simulink model "MODEL_FULL_SYSTEM_MUTUAL"  (Simulink 7.8)
settings: Solver=ode1  StartTime=0.0  StopTime=inf  FixedStep=Ts  MaxStep=1e-3  RelTol=1e-3
PostLoadFcn:
  | Ts=80e-6; relays_settings_init;
InitFcn:
  | Ts=80e-6; relays_settings_init;
values from neighbouring files (symbols this model uses):
  relay_sets = xlsread('relay_settings_10272015.xlsx')    [relays_settings_init.m]
undefined symbols (not defined in the file or in its folder): dfilt, DiscIntNeverNeededParam, fdesignblkfcn, gcbh, Left, opmodbus_cb, ph, Right, type, V, X
libraries: simulink x72, modbus_lib x40, cables_lib x36, rtio_opalrt_common x21, rtlab x20, transformer_lib x13, dynamic_load_lib x12, powerlib x6, simulink_extras x6, ssn_lib x5, discretizing x4, rteventslib x4
(part 4 of 7)

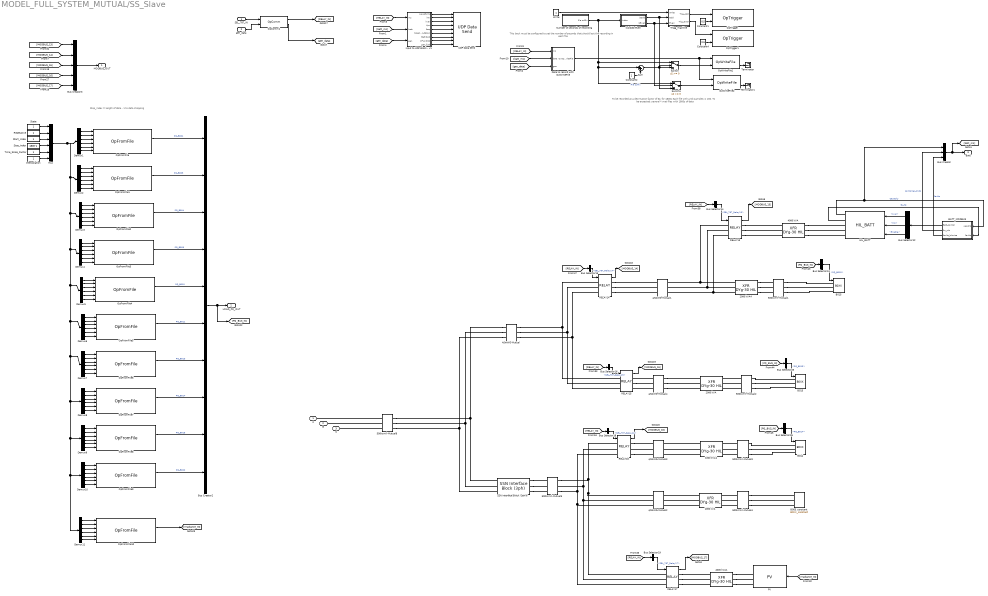
== system MODEL_FULL_SYSTEM_MUTUAL/SS_Slave ==
  note: Stop_index = length of data - 1 to data chopping
  note: This bock must be configured to set the number of
      | seconds that should last the recording in each file
  note: To be recorded at a decimation factor of 62,   for 1800s each file with a Nb samples = 200.
      | To be expected: several *.mat files with 1800s of data
  SEL_787_IN : Inport
  gen_data : Inport  Port=2
  1000 kVA : transformer_lib/XFR DYg-30 HIL  Rating=1000  Vp=4160  Vs=460  Z=5.18  XR=2.5
  1000 kVA1 : transformer_lib/XFR DYg-30 HIL  Rating=1000  Vp=4160  Vs=216  Z=5.18  XR=2.5
  2000 kVA : transformer_lib/XFR DYg-30 HIL  Rating=2000  Vp=4160  Vs=216  Z=5.18  XR=2.5
  2000 kVA4 : transformer_lib/XFR DYg-30 HIL  Rating=2000  Vp=4160  Vs=216  Z=5.18  XR=2.5
  4/0AWG-Mutual : cables_lib/4//0AWG-Mutual  length=20  par_sets=1  ratio=3
  4/0AWG-Mutual{1..4} (4 alike) : cables_lib/4//0AWG-Mutual  length=51  par_sets=1  ratio=3
  4000 kVA : transformer_lib/XFR DYg-30 HIL  Rating=4000  Vp=2047  Vs=4160  Z=6.37  XR=3.5
  4000 kVA1 : transformer_lib/XFR DYg-30 HIL  Rating=4000  Vp=2047  Vs=4160  Z=6.37  XR=3.5
  500kcmil-Mutual{1..4} (4 alike) : cables_lib/500kcmil-Mutual  length=25  par_sets=1  ratio=3
  500kcmil-Mutual5 : cables_lib/500kcmil-Mutual  length=50  par_sets=1  ratio=3
  500kcmil-Mutual8 : cables_lib/500kcmil-Mutual  length=50  par_sets=1  ratio=3
  B003_constant : dynamic_load_lib/B0XX_constant  v=460  kVA=60  pf=0.9
  B013 : dynamic_load_lib/B0XX  V=208  P_Scale=2  Q_Scale=2
  B014 : dynamic_load_lib/B0XX  V=208  P_Scale=1  Q_Scale=1
  B015 : dynamic_load_lib/B0XX  V=208  P_Scale=2  Q_Scale=2
  BATT_MODBUS : Subsystem
  Bus Creator : BusCreator  Inputs=3
  Bus Creator2 : BusCreator  Inputs=10
  Bus Creator3 : BusCreator  Inputs=5
  Bus Selector12 : BusSelector  OutputSignals=kvar,kW,Enable
  Bus Selector14 : BusSelector  OutputSignals=SEL_787_Relay13
  Bus Selector15 : BusSelector  OutputSignals=SEL_787_Relay14
  Bus Selector16 : BusSelector  OutputSignals=SEL_787_Relay15
  Bus Selector18 : BusSelector  OutputSignals=SEL_787_Relay16
  Bus Selector19 : BusSelector  OutputSignals=SEL_787_Relay17
  Bus Selector24 : BusSelector  OutputSignals=PQ_B015
  Bus Selector25 : BusSelector  OutputSignals=PQ_B013
  Bus Selector26 : BusSelector  OutputSignals=PQ_B014
  Constant1 : Constant  Value=0.5
  Constant2 : Constant
  Constant4 : Constant  Value=0.5
  Data to record with OpWriteFile : Subsystem
  Demux{1..11} (11 alike) : Demux  Outputs=6
  HIL_BATT : Batt_lib/HIL_BATT
  Input to UDP Block - v1 : Subsystem
  "Interpolation " : Constant
  Mux : Mux  Inputs=6
  Number of seconds of recording : Subsystem  mask{time_s=1800}
      mask prompts: time_s "Time in seconds"
      mask help: Set the number of seconds that should last the recording in each file.
  OpComm1 : rtlab/OpComm  nbport=2  groupe_acq=1  subsys_rate=0  st=0  Synchronization=on  Interpolation=on  Threshold=1.0  Missed_Data=off  Sim_Time=off  Samples=off  dynSigOut=off  from_console=0  warning_done=off  writeOpCommFile=off  Offset=off
  OpFromFile : rtlab/DataLogging/OpFromFile  filename_mode=Static (same filename all the time)  reload_mode=Next time model is paused (Real-Time)  init_file_id=0  filename=B001.mat  rtpath='./'  nrtpath='.\'  sample_time=0
  OpFromFile1 : rtlab/DataLogging/OpFromFile  filename_mode=Static (same filename all the time)  reload_mode=Next time model is paused (Real-Time)  init_file_id=0  filename=B003.mat  rtpath='./'  nrtpath='.\'  sample_time=0
  OpFromFile10 : rtlab/DataLogging/OpFromFile  filename_mode=Static (same filename all the time)  reload_mode=Next time model is paused (Real-Time)  init_file_id=0  filename=irradiance_data.mat  rtpath='./'  nrtpath='.\'  sample_time=Ts
  OpFromFile2 : rtlab/DataLogging/OpFromFile  filename_mode=Static (same filename all the time)  reload_mode=Next time model is paused (Real-Time)  init_file_id=0  filename=B004.mat  rtpath='./'  nrtpath='.\'  sample_time=0
  OpFromFile3 : rtlab/DataLogging/OpFromFile  filename_mode=Static (same filename all the time)  reload_mode=Next time model is paused (Real-Time)  init_file_id=0  filename=B009.mat  rtpath='./'  nrtpath='.\'  sample_time=0
  OpFromFile4 : rtlab/DataLogging/OpFromFile  filename_mode=Static (same filename all the time)  reload_mode=Next time model is paused (Real-Time)  init_file_id=0  filename=B010.mat  rtpath='./'  nrtpath='.\'  sample_time=0
  OpFromFile5 : rtlab/DataLogging/OpFromFile  filename_mode=Static (same filename all the time)  reload_mode=Next time model is paused (Real-Time)  init_file_id=0  filename=B011.mat  rtpath='./'  nrtpath='.\'  sample_time=0
  OpFromFile6 : rtlab/DataLogging/OpFromFile  filename_mode=Static (same filename all the time)  reload_mode=Next time model is paused (Real-Time)  init_file_id=0  filename=B013.mat  rtpath='./'  nrtpath='.\'  sample_time=0
  OpFromFile7 : rtlab/DataLogging/OpFromFile  filename_mode=Static (same filename all the time)  reload_mode=Next time model is paused (Real-Time)  init_file_id=0  filename=B014.mat  rtpath='./'  nrtpath='.\'  sample_time=0
  OpFromFile8 : rtlab/DataLogging/OpFromFile  filename_mode=Static (same filename all the time)  reload_mode=Next time model is paused (Real-Time)  init_file_id=0  filename=B015.mat  rtpath='./'  nrtpath='.\'  sample_time=0
  OpFromFile9 : rtlab/DataLogging/OpFromFile  filename_mode=Static (same filename all the time)  reload_mode=Next time model is paused (Real-Time)  init_file_id=0  filename=B022.mat  rtpath='./'  nrtpath='.\'  sample_time=0
  OpTrigger : rtlab/DataLogging/OpTrigger  Trig_Type=TRIGGER SIGNAL >= TRIGGER LEVEL  Trig_Offset=0  Acq_Group=28
  OpTrigger1 : rtlab/DataLogging/OpTrigger  Trig_Type=TRIGGER SIGNAL >= TRIGGER LEVEL  Trig_Offset=0  Acq_Group=29
  OpWriteFile1 : rtlab/DataLogging/OpWriteFile  Static_File=off  varname=recVar  Filename=A_FILE_RECORDED_o.mat  rtpath='./'  nrtpath='.\'  Acq_Group=28  file_size=200000000  write_offline=off  Sim_Mode=off  Nb_Samples=200  Buffer_size=0
      settings: Decimation=62
  OpWriteFile2 : rtlab/DataLogging/OpWriteFile  Static_File=off  varname=recVar  Filename=A_FILE_RECORDED_e.mat  rtpath='./'  nrtpath='.\'  Acq_Group=29  file_size=200000000  write_offline=on  Sim_Mode=off  Nb_Samples=200  Buffer_size=0
      settings: Decimation=62
  PV : PV_lib/PV  max_power=4e6  VacRMS=1200  VacRMS_limit_pu=[1.15 0.85]
  RELAY13 : modbus_lib/RELAY  Ts=Ts
      link override Three-Phase V-I Measurement/Model/VI/Ia: GotoTag=LibraryTag_Ia
      link override Three-Phase V-I Measurement/Model/VI/Ib: GotoTag=LibraryTag_Ib
      link override Three-Phase V-I Measurement/Model/VI/Ic: GotoTag=LibraryTag_Ic
      link override Three-Phase V-I Measurement/Model/VI/Va: GotoTag=LibraryTag_Va
      link override Three-Phase V-I Measurement/Model/VI/Vb: GotoTag=LibraryTag_Vb
      link override Three-Phase V-I Measurement/Model/VI/Vc: GotoTag=LibraryTag_Vc
      link override Three-Phase V-I Measurement1/Model/VI/Ia: GotoTag=LibraryTag_Ia
      link override Three-Phase V-I Measurement1/Model/VI/Ib: GotoTag=LibraryTag_Ib
      link override Three-Phase V-I Measurement1/Model/VI/Ic: GotoTag=LibraryTag_Ic
      link override Three-Phase V-I Measurement1/Model/VI/Va: GotoTag=LibraryTag_Va
      link override Three-Phase V-I Measurement1/Model/VI/Vb: GotoTag=LibraryTag_Vb
      link override Three-Phase V-I Measurement1/Model/VI/Vc: GotoTag=LibraryTag_Vc
  RELAY14 : modbus_lib/RELAY  Ts=Ts
      link override Three-Phase V-I Measurement/Model/VI/Ia: GotoTag=LibraryTag_Ia
      link override Three-Phase V-I Measurement/Model/VI/Ib: GotoTag=LibraryTag_Ib
      link override Three-Phase V-I Measurement/Model/VI/Ic: GotoTag=LibraryTag_Ic
      link override Three-Phase V-I Measurement/Model/VI/Va: GotoTag=LibraryTag_Va
      link override Three-Phase V-I Measurement/Model/VI/Vb: GotoTag=LibraryTag_Vb
      link override Three-Phase V-I Measurement/Model/VI/Vc: GotoTag=LibraryTag_Vc
      link override Three-Phase V-I Measurement1/Model/VI/Ia: GotoTag=LibraryTag_Ia
      link override Three-Phase V-I Measurement1/Model/VI/Ib: GotoTag=LibraryTag_Ib
      link override Three-Phase V-I Measurement1/Model/VI/Ic: GotoTag=LibraryTag_Ic
      link override Three-Phase V-I Measurement1/Model/VI/Va: GotoTag=LibraryTag_Va
      link override Three-Phase V-I Measurement1/Model/VI/Vb: GotoTag=LibraryTag_Vb
      link override Three-Phase V-I Measurement1/Model/VI/Vc: GotoTag=LibraryTag_Vc
  RELAY15 : modbus_lib/RELAY  Ts=Ts
      link override Three-Phase V-I Measurement/Model/VI/Ia: GotoTag=LibraryTag_Ia
      link override Three-Phase V-I Measurement/Model/VI/Ib: GotoTag=LibraryTag_Ib
      link override Three-Phase V-I Measurement/Model/VI/Ic: GotoTag=LibraryTag_Ic
      link override Three-Phase V-I Measurement/Model/VI/Va: GotoTag=LibraryTag_Va
      link override Three-Phase V-I Measurement/Model/VI/Vb: GotoTag=LibraryTag_Vb
      link override Three-Phase V-I Measurement/Model/VI/Vc: GotoTag=LibraryTag_Vc
      link override Three-Phase V-I Measurement1/Model/VI/Ia: GotoTag=LibraryTag_Ia
      link override Three-Phase V-I Measurement1/Model/VI/Ib: GotoTag=LibraryTag_Ib
      link override Three-Phase V-I Measurement1/Model/VI/Ic: GotoTag=LibraryTag_Ic
      link override Three-Phase V-I Measurement1/Model/VI/Va: GotoTag=LibraryTag_Va
      link override Three-Phase V-I Measurement1/Model/VI/Vb: GotoTag=LibraryTag_Vb
      link override Three-Phase V-I Measurement1/Model/VI/Vc: GotoTag=LibraryTag_Vc
  RELAY16 : modbus_lib/RELAY  Ts=Ts
      link override Three-Phase V-I Measurement/Model/VI/Ia: GotoTag=LibraryTag_Ia
      link override Three-Phase V-I Measurement/Model/VI/Ib: GotoTag=LibraryTag_Ib
      link override Three-Phase V-I Measurement/Model/VI/Ic: GotoTag=LibraryTag_Ic
      link override Three-Phase V-I Measurement/Model/VI/Va: GotoTag=LibraryTag_Va
      link override Three-Phase V-I Measurement/Model/VI/Vb: GotoTag=LibraryTag_Vb
      link override Three-Phase V-I Measurement/Model/VI/Vc: GotoTag=LibraryTag_Vc
      link override Three-Phase V-I Measurement1/Model/VI/Ia: GotoTag=LibraryTag_Ia
      link override Three-Phase V-I Measurement1/Model/VI/Ib: GotoTag=LibraryTag_Ib
      link override Three-Phase V-I Measurement1/Model/VI/Ic: GotoTag=LibraryTag_Ic
      link override Three-Phase V-I Measurement1/Model/VI/Va: GotoTag=LibraryTag_Va
      link override Three-Phase V-I Measurement1/Model/VI/Vb: GotoTag=LibraryTag_Vb
      link override Three-Phase V-I Measurement1/Model/VI/Vc: GotoTag=LibraryTag_Vc
  RELAY17 : modbus_lib/RELAY  Ts=Ts
      link override Three-Phase V-I Measurement/Model/VI/Ia: GotoTag=LibraryTag_Ia
      link override Three-Phase V-I Measurement/Model/VI/Ib: GotoTag=LibraryTag_Ib
      link override Three-Phase V-I Measurement/Model/VI/Ic: GotoTag=LibraryTag_Ic
      link override Three-Phase V-I Measurement/Model/VI/Va: GotoTag=LibraryTag_Va
      link override Three-Phase V-I Measurement/Model/VI/Vb: GotoTag=LibraryTag_Vb
      link override Three-Phase V-I Measurement/Model/VI/Vc: GotoTag=LibraryTag_Vc
      link override Three-Phase V-I Measurement1/Model/VI/Ia: GotoTag=LibraryTag_Ia
      link override Three-Phase V-I Measurement1/Model/VI/Ib: GotoTag=LibraryTag_Ib
      link override Three-Phase V-I Measurement1/Model/VI/Ic: GotoTag=LibraryTag_Ic
      link override Three-Phase V-I Measurement1/Model/VI/Va: GotoTag=LibraryTag_Va
      link override Three-Phase V-I Measurement1/Model/VI/Vb: GotoTag=LibraryTag_Vb
      link override Three-Phase V-I Measurement1/Model/VI/Vc: GotoTag=LibraryTag_Vc
  "Repetative " : Constant
  SSN Interface Block (3ph)6 : ssn_lib/SSN Interface Block (3ph)  nb_phase=3  nb_port=2  p1_type=V-type(Left)  p2_type=V-type (Right)  p3_type=V-type (Right)  p4_type=V-type(Left)  p5_type=V-type(Left)  p6_type=V-type(Left)  p7_type=V-type(Left)  p8_type=V-type(Left)  p9_type=V-type(Left)  p10_type=V-type(Left)  p11_type=V-type(Left)  p12_type=V-type(Left)  p13_type=V-type(Left)  p14_type=V-type(Left)  p15_type=V-type(Left)  p16_type=V-type(Left)  I_port_shunt_resistance=1e9
  "Start_Index " : Constant
  "State " : Constant
  "Stop_Index " : Constant  Value=1800-1
  Sum : Sum  Inputs=|++
  Switch : Switch
  Switch1 : Switch
  Terminator : Terminator
  Terminator1 : Terminator
  "Time_Scale_Factor " : Constant
  Trigg_machine : Subsystem
  UDP Data Send : HIL_UDP_lib/UDP Data Send
  Write : Constant
  isOddOrEven : Subsystem
  A : PMIOPort  Port=1  Side=Left
  B : PMIOPort  Port=2  Side=Left
  C : PMIOPort  Port=3  Side=Left
  MODBUS_OUT : Outport
  LOAD_PQ_OUT : Outport  Port=2
  Batt : Outport  Port=3
  wires:
  [Irradiance_IN] -> PV/1
  Bus Selector26/1 -> B014/1  "<PQ_B014>"
  [PQ_BUS_IN] -> Bus Selector26/1
  Bus Selector25/1 -> B013/1  "<PQ_B013>"
  [PQ_BUS_IN] -> Bus Selector25/1
  Bus Selector24/1 -> B015/1  "<PQ_B015>"
  [PQ_BUS_IN] -> Bus Selector24/1
  [RELAY_IN] -> Bus Selector19/1
  Bus Selector18/1 -> RELAY16/1  "<SEL_787_Relay16>"
  [RELAY_IN] -> Bus Selector18/1
  Bus Selector16/1 -> RELAY15/1  "<SEL_787_Relay15>"
  [RELAY_IN] -> Bus Selector16/1
  Bus Selector15/1 -> RELAY14/1  "<SEL_787_Relay14>"
  [RELAY_IN] -> Bus Selector15/1
  [RELAY_IN] -> Bus Selector14/1
  RELAY16/1 -> [MODBUS_16]
  RELAY15/1 -> [MODBUS_15]
  RELAY14/1 -> [MODBUS_14]
  SEL_787_IN/1 -> OpComm1/1
  OpComm1/1 -> [RELAY_IN]
  Bus Creator3/1 -> MODBUS_OUT/1
  Demux1/6 -> OpFromFile/6
  Demux1/5 -> OpFromFile/5
  Demux1/4 -> OpFromFile/4
  Demux1/3 -> OpFromFile/3
  Demux1/2 -> OpFromFile/2
  Demux1/1 -> OpFromFile/1
  Mux/1 -> Demux1/1, Demux2/1, Demux3/1, Demux4/1, Demux5/1, Demux6/1, Demux7/1, Demux8/1, Demux9/1, Demux10/1, Demux11/1
  "Interpolation "/1 -> Mux/6
  "Time_Scale_Factor "/1 -> Mux/5
  "Stop_Index "/1 -> Mux/4
  "Start_Index "/1 -> Mux/3
  "Repetative "/1 -> Mux/2
  "State "/1 -> Mux/1
  OpFromFile/2 -> Bus Creator2/1  "PQ_B001"
  Demux2/6 -> OpFromFile1/6
  Demux2/5 -> OpFromFile1/5
  Demux2/4 -> OpFromFile1/4
  Demux2/3 -> OpFromFile1/3
  Demux2/2 -> OpFromFile1/2
  Demux2/1 -> OpFromFile1/1
  OpFromFile1/2 -> Bus Creator2/2  "PQ_B003"
  Demux3/6 -> OpFromFile2/6
  Demux3/5 -> OpFromFile2/5
  Demux3/4 -> OpFromFile2/4
  Demux3/3 -> OpFromFile2/3
  Demux3/2 -> OpFromFile2/2
  Demux3/1 -> OpFromFile2/1
  OpFromFile2/2 -> Bus Creator2/3  "PQ_B004"
  Demux4/6 -> OpFromFile3/6
  Demux4/5 -> OpFromFile3/5
  Demux4/4 -> OpFromFile3/4
  Demux4/3 -> OpFromFile3/3
  Demux4/2 -> OpFromFile3/2
  Demux4/1 -> OpFromFile3/1
  OpFromFile3/2 -> Bus Creator2/4  "PQ_B009"
  Demux5/6 -> OpFromFile4/6
  Demux5/5 -> OpFromFile4/5
  Demux5/4 -> OpFromFile4/4
  Demux5/3 -> OpFromFile4/3
  Demux5/2 -> OpFromFile4/2
  Demux5/1 -> OpFromFile4/1
  OpFromFile4/2 -> Bus Creator2/5  "PQ_B010"
  Demux6/6 -> OpFromFile5/6
  Demux6/5 -> OpFromFile5/5
  Demux6/4 -> OpFromFile5/4
  Demux6/3 -> OpFromFile5/3
  Demux6/2 -> OpFromFile5/2
  Demux6/1 -> OpFromFile5/1
  OpFromFile5/2 -> Bus Creator2/6  "PQ_B011"
  Demux7/6 -> OpFromFile6/6
  Demux7/5 -> OpFromFile6/5
  Demux7/4 -> OpFromFile6/4
  Demux7/3 -> OpFromFile6/3
  Demux7/2 -> OpFromFile6/2
  Demux7/1 -> OpFromFile6/1
  OpFromFile6/2 -> Bus Creator2/7  "PQ_B013"
  Demux8/6 -> OpFromFile7/6
  Demux8/5 -> OpFromFile7/5
  Demux8/4 -> OpFromFile7/4
  Demux8/3 -> OpFromFile7/3
  Demux8/2 -> OpFromFile7/2
  Demux8/1 -> OpFromFile7/1
  OpFromFile7/2 -> Bus Creator2/8  "PQ_B014"
  Demux9/6 -> OpFromFile8/6
  Demux9/5 -> OpFromFile8/5
  Demux9/4 -> OpFromFile8/4
  Demux9/3 -> OpFromFile8/3
  Demux9/2 -> OpFromFile8/2
  Demux9/1 -> OpFromFile8/1
  OpFromFile8/2 -> Bus Creator2/9  "PQ_B015"
  Demux10/6 -> OpFromFile9/6
  Demux10/5 -> OpFromFile9/5
  Demux10/4 -> OpFromFile9/4
  Demux10/3 -> OpFromFile9/3
  Demux10/2 -> OpFromFile9/2
  Demux10/1 -> OpFromFile9/1
  OpFromFile9/2 -> Bus Creator2/10  "PQ_B022"
  Bus Creator2/1 -> LOAD_PQ_OUT/1, [PQ_BUS_IN]
  Demux11/1 -> OpFromFile10/1
  Demux11/2 -> OpFromFile10/2
  Demux11/3 -> OpFromFile10/3
  Demux11/4 -> OpFromFile10/4
  Demux11/5 -> OpFromFile10/5
  Demux11/6 -> OpFromFile10/6
  OpFromFile10/2 -> [Irradiance_IN]
  BATT_MODBUS/1(Batt_control) -> Bus Selector12/1
  Bus Selector19/1 -> RELAY17/1  "<SEL_787_Relay17>"
  RELAY17/1 -> [MODBUS_17]
  Bus Selector14/1 -> RELAY13/1  "<SEL_787_Relay13>"
  RELAY13/1 -> [MODBUS_13]
  Bus Creator/1 -> Batt/1, [batt_ms]
  BATT_MODBUS/2(fm_mb) -> Bus Creator/2  "controller_cmds"
  HIL_BATT/2 -> BATT_MODBUS/2(faults)  "faults"
  HIL_BATT/1 -> BATT_MODBUS/1(MSMTS), Bus Creator/1  "Capacity"
  BATT_MODBUS/3(faults_bitwise) -> Bus Creator/3  "faults"
  [batt_ms] -> Data to record with OpWriteFile/2(batt)
  [gen_data] -> Data to record with OpWriteFile/3(gen)
  gen_data/1 -> OpComm1/2
  OpComm1/2 -> [gen_data]
  [RELAY_IN] -> Data to record with OpWriteFile/1(ms)
  Bus Selector12/1 -> HIL_BATT/1  "<kvar>"
  Bus Selector12/2 -> HIL_BATT/2  "<kW>"
  Bus Selector12/3 -> HIL_BATT/3  "<Enable>"
  Input to UDP Block - v1/1(waveforms) -> UDP Data Send/1
  Input to UDP Block - v1/2(kW) -> UDP Data Send/2
  Input to UDP Block - v1/3(kvar) -> UDP Data Send/3
  Input to UDP Block - v1/4(Vpu) -> UDP Data Send/4
  Input to UDP Block - v1/5(freq) -> UDP Data Send/5
  Input to UDP Block - v1/6(breaker_status) -> UDP Data Send/6
  Input to UDP Block - v1/7(Batt SoC) -> UDP Data Send/7
  Input to UDP Block - v1/8(PF at PCC) -> UDP Data Send/8
  [RELAY_IN] -> Input to UDP Block - v1/1(ms)
  [batt_ms] -> Input to UDP Block - v1/2(batt)
  [gen_data] -> Input to UDP Block - v1/3(gen)
  Input to UDP Block - v1/9(gen_fuel) -> UDP Data Send/9
  Data to record with OpWriteFile/1(to OpWriteFile) -> OpWriteFile2/1, OpWriteFile1/1
  Trigg_machine/1(Trig_odd) -> OpTrigger/1
  Trigg_machine/2(Trig_even) -> OpTrigger1/1
  Constant1/1 -> OpTrigger/2
  Constant4/1 -> OpTrigger1/2
  isOddOrEven/1(isOdd) -> Switch/2, Trigg_machine/2(Odd)
  isOddOrEven/2(isEven) -> Switch1/2, Trigg_machine/3(Even)
  Switch/1 -> OpWriteFile1/2
  Switch1/1 -> OpWriteFile2/2
  Constant2/1 -> Sum/2
  Sum/1 -> Switch/3, Switch1/3
  Number of seconds of recording/1(file suffix) -> isOddOrEven/1(Index), Sum/1, Switch1/1, Switch/1  "File suffix"
  Write/1 -> Trigg_machine/1(Write)
  OpWriteFile1/2 -> Terminator/1
  OpWriteFile2/2 -> Terminator1/1
  [MODBUS_13] -> Bus Creator3/1
  [MODBUS_14] -> Bus Creator3/2
  [MODBUS_15] -> Bus Creator3/3
  [MODBUS_16] -> Bus Creator3/4
  [MODBUS_17] -> Bus Creator3/5
  connections:
  500kcmil-Mutual4/RConn3 -- B003_constant/LConn3
  500kcmil-Mutual4/RConn2 -- B003_constant/LConn2
  500kcmil-Mutual4/RConn1 -- B003_constant/LConn1
  RELAY16/RConn3 -- 4/0AWG-Mutual3/LConn3
  4/0AWG-Mutual3/LConn2 -- RELAY16/RConn2
  RELAY16/RConn1 -- 4/0AWG-Mutual3/LConn1
  4/0AWG-Mutual4/LConn3 -- RELAY15/RConn3
  RELAY15/RConn2 -- 4/0AWG-Mutual4/LConn2
  4/0AWG-Mutual4/LConn1 -- RELAY15/RConn1
  4/0AWG-Mutual/RConn3 -- RELAY15/LConn3 -- RELAY14/LConn3
  4/0AWG-Mutual/RConn2 -- RELAY15/LConn2 -- RELAY14/LConn2
  4/0AWG-Mutual/RConn1 -- RELAY15/LConn1 -- RELAY14/LConn1
  4/0AWG-Mutual2/LConn3 -- RELAY17/LConn3 -- RELAY16/LConn3 -- 500kcmil-Mutual5/RConn3
  4/0AWG-Mutual2/LConn1 -- RELAY17/LConn1 -- RELAY16/LConn1 -- 500kcmil-Mutual5/RConn1
  2000 kVA4/RConn3 -- 500kcmil-Mutual1/LConn3
  2000 kVA4/RConn2 -- 500kcmil-Mutual1/LConn2
  2000 kVA4/RConn1 -- 500kcmil-Mutual1/LConn1
  4/0AWG-Mutual1/RConn3 -- RELAY13/LConn3 -- 2000 kVA4/LConn3
  4/0AWG-Mutual1/RConn2 -- RELAY13/LConn2 -- 2000 kVA4/LConn2
  4/0AWG-Mutual1/RConn1 -- RELAY13/LConn1 -- 2000 kVA4/LConn1
  500kcmil-Mutual2/LConn3 -- 2000 kVA/RConn3
  500kcmil-Mutual2/LConn2 -- 2000 kVA/RConn2
  500kcmil-Mutual2/LConn1 -- 2000 kVA/RConn1
  4/0AWG-Mutual4/RConn3 -- 2000 kVA/LConn3
  4/0AWG-Mutual4/RConn2 -- 2000 kVA/LConn2
  4/0AWG-Mutual4/RConn1 -- 2000 kVA/LConn1
  500kcmil-Mutual3/LConn3 -- 1000 kVA1/RConn3
  500kcmil-Mutual3/LConn2 -- 1000 kVA1/RConn2
  500kcmil-Mutual3/LConn1 -- 1000 kVA1/RConn1
  1000 kVA1/LConn3 -- 4/0AWG-Mutual3/RConn3
  1000 kVA1/LConn2 -- 4/0AWG-Mutual3/RConn2
  1000 kVA1/LConn1 -- 4/0AWG-Mutual3/RConn1
  500kcmil-Mutual4/LConn3 -- 1000 kVA/RConn3
  500kcmil-Mutual4/LConn2 -- 1000 kVA/RConn2
  500kcmil-Mutual4/LConn1 -- 1000 kVA/RConn1
  1000 kVA/LConn3 -- 4/0AWG-Mutual2/RConn3
  1000 kVA/LConn2 -- 4/0AWG-Mutual2/RConn2
  1000 kVA/LConn1 -- 4/0AWG-Mutual2/RConn1
  RELAY17/RConn3 -- 4000 kVA1/RConn3
  RELAY17/RConn2 -- 4000 kVA1/RConn2
  RELAY17/RConn1 -- 4000 kVA1/RConn1
  RELAY13/RConn3 -- 4000 kVA/RConn3
  RELAY13/RConn2 -- 4000 kVA/RConn2
  RELAY13/RConn1 -- 4000 kVA/RConn1
  500kcmil-Mutual8/LConn1 -- A/RConn1
  500kcmil-Mutual8/LConn2 -- B/RConn1
  500kcmil-Mutual8/LConn3 -- C/RConn1
  500kcmil-Mutual3/RConn3 -- B014/LConn3
  500kcmil-Mutual3/RConn2 -- B014/LConn2
  500kcmil-Mutual3/RConn1 -- B014/LConn1
  500kcmil-Mutual2/RConn3 -- B013/LConn3
  500kcmil-Mutual2/RConn2 -- B013/LConn2
  500kcmil-Mutual2/RConn1 -- B013/LConn1
  500kcmil-Mutual1/RConn3 -- B015/LConn3
  500kcmil-Mutual1/RConn2 -- B015/LConn2
  500kcmil-Mutual1/RConn1 -- B015/LConn1
  RELAY14/RConn3 -- 4/0AWG-Mutual1/LConn3
  RELAY14/RConn2 -- 4/0AWG-Mutual1/LConn2
  RELAY14/RConn1 -- 4/0AWG-Mutual1/LConn1
  4/0AWG-Mutual2/LConn2 -- RELAY17/LConn2 -- RELAY16/LConn2 -- 500kcmil-Mutual5/RConn2
  4000 kVA1/LConn3 -- PV/RConn3
  4000 kVA1/LConn2 -- PV/RConn2
  4000 kVA1/LConn1 -- PV/RConn1
  4000 kVA/LConn3 -- HIL_BATT/RConn3
  4000 kVA/LConn2 -- HIL_BATT/RConn2
  4000 kVA/LConn1 -- HIL_BATT/RConn1
  4/0AWG-Mutual/LConn3 -- SSN Interface Block (3ph)6/LConn3 -- 500kcmil-Mutual8/RConn3
  4/0AWG-Mutual/LConn2 -- SSN Interface Block (3ph)6/LConn2 -- 500kcmil-Mutual8/RConn2
  4/0AWG-Mutual/LConn1 -- SSN Interface Block (3ph)6/LConn1 -- 500kcmil-Mutual8/RConn1
  SSN Interface Block (3ph)6/RConn3 -- 500kcmil-Mutual5/LConn3
  SSN Interface Block (3ph)6/RConn2 -- 500kcmil-Mutual5/LConn2
  SSN Interface Block (3ph)6/RConn1 -- 500kcmil-Mutual5/LConn1

== system MODEL_FULL_SYSTEM_MUTUAL/SC_Console/Woodward2 ==
  note: Op_Mode:
      | 0 = Relay Functions
      | 1 = Close Breaker
      | 2 = Open Breaker
  note: This corresponds to
      | the DIO Enable MCB
  Gen1_Primary : Inport
  Gen2_Primary : Inport  Port=2
  DIn_Ch00_31 : Inport  Port=3
  16Din/16Dout GR3 : Subsystem
  16PWMIn/16PWMout GR3 : Subsystem
  16TSDIn/16 TSDOut GR3 : Subsystem
  Brk1 Grid : Constant  Value=2
  Brk10 Gen 1 Busbar : Constant
  Brk2 Load 1 : Constant  Value=0
  Brk3 Gen 2 MCB : Constant  Value=2
  Brk4 Gen 1 MCB : Constant  Value=2
  Brk5 Gen 2 LCB : Constant  Value=0
  Brk6 Gen 1 LCB : Constant  Value=0
  Brk7 Gen 2 GCB : Constant
  Brk8 Gen 1 GCB : Constant
  Brk9 Gen 2 Busbar : Constant
  Bus Creator{1..2,4..5} (4 alike) : BusCreator  Inputs=3
  Bus Creator3 : BusCreator  Inputs=14
  Bus Selector1 : BusSelector  OutputSignals=Pm,Vf,Vt,w
  Bus Selector2 : BusSelector  OutputSignals=Pm,Vf,Vt,w
  Bus Selector3 : BusSelector  OutputSignals="signal1,w.wood_Gov_bias,w.Rotor speed  wm (pu)"
  Bus Selector4 : BusSelector  OutputSignals="signal1,w.wood_Gov_bias,w.Rotor speed  wm (pu)"
  Gain : Gain  Gain=10
  Gain1 : Gain  Gain=10
  Scope_Gen1_Primary : Scope  NumInputPorts=4
      settings: TimeRange=60  YMin=0~-5~-1~-1  YMax=1.1~5~2~2  SaveName=ScopeData4
  Scope_Gen2_Primary : Scope  NumInputPorts=4
      settings: TimeRange=60  YMin=0~-5~-1~-1  YMax=1.1~5~2~2  SaveName=ScopeData3
  Wood MCB Enable : Constant  Value=0
  bias_ctrl : Constant
  control mode 1 for Woodward 0 for simulation 1 : Constant  Value=0
  control_mode : Constant
  gen_enable : Constant
  Out1 : Outport
  wires:
  control mode 1 for Woodward 0 for simulation 1/1 -> Bus Creator2/1  "Woodward"
  16Din/16Dout GR3/1(Dout) -> Bus Creator1/1  "16 DOUT GR3"
  16TSDIn/16 TSDOut GR3/1(TSDout) -> Bus Creator1/2  "16 TSDOUT GR3"
  16PWMIn/16PWMout GR3/1(To PWMOut) -> Bus Creator1/3  "16 PWMOUT GR3"
  Bus Creator1/1 -> Bus Creator2/3  "DOUT GR3"
  Bus Creator3/1 -> Bus Creator2/2  "test_controls"
  Brk1 Grid/1 -> Bus Creator3/1  "Grid"
  Brk2 Load 1/1 -> Bus Creator3/2  "Load 1"
  Brk3 Gen 2 MCB/1 -> Bus Creator3/3  "Gen2_MCB"
  Brk4 Gen 1 MCB/1 -> Bus Creator3/4  "Gen1_MCB"
  control_mode/1 -> Bus Creator3/11  "Wood_DIO"
  gen_enable/1 -> Bus Creator3/12  "Gen2_enable"
  bias_ctrl/1 -> Bus Creator3/13  "Gen_bias_enable"
  Bus Creator2/1 -> Out1/1
  DIn_Ch00_31/1 -> 16Din/16Dout GR3/1(Din)
  Bus Selector1/1 -> Scope_Gen1_Primary/1  "<Pm>"
  Bus Selector1/2 -> Scope_Gen1_Primary/2  "<Vf>"
  Bus Selector1/3 -> Scope_Gen1_Primary/3  "<Vt>"
  Gen1_Primary/1 -> Bus Selector1/1
  Wood MCB Enable/1 -> Bus Creator3/14  "Wood_MCB_enable"
  Gen2_Primary/1 -> Bus Selector2/1
  Bus Selector2/1 -> Scope_Gen2_Primary/1  "<Pm>"
  Bus Selector2/2 -> Scope_Gen2_Primary/2  "<Vf>"
  Bus Selector2/3 -> Scope_Gen2_Primary/3  "<Vt>"
  Bus Selector1/4 -> Bus Selector3/1  "<w>"
  Bus Selector3/1 -> Bus Creator4/1  "<signal1>"
  Bus Selector3/2 -> Gain/1  "<wood_Gov_bias>"
  Bus Selector3/3 -> Bus Creator4/3  "<Rotor speed  wm (pu)>"
  Bus Creator4/1 -> Scope_Gen1_Primary/4
  Bus Selector4/1 -> Bus Creator5/1  "<signal1>"
  Bus Selector4/2 -> Gain1/1  "<wood_Gov_bias>"
  Bus Selector4/3 -> Bus Creator5/3  "<Rotor speed  wm (pu)>"
  Bus Selector2/4 -> Bus Selector4/1  "<w>"
  Bus Creator5/1 -> Scope_Gen2_Primary/4
  Brk5 Gen 2 LCB/1 -> Bus Creator3/5  "Load 2"
  Brk6 Gen 1 LCB/1 -> Bus Creator3/6  "Load 3"
  Brk7 Gen 2 GCB/1 -> Bus Creator3/7  "Gen2_GCB"
  Brk8 Gen 1 GCB/1 -> Bus Creator3/8  "Gen1_GCB"
  Gain1/1 -> Bus Creator5/2
  Gain/1 -> Bus Creator4/2
  Brk9 Gen 2 Busbar/1 -> Bus Creator3/9  "Gen2_Busbar"
  Brk10 Gen 1 Busbar/1 -> Bus Creator3/10  "Gen1_Busbar"

== system MODEL_FULL_SYSTEM_MUTUAL/SC_Console/system-overall ==
  ms : Inport
  Bus Selector10 : BusSelector  OutputSignals=SEL_787_Relay1.m.Vpu,SEL_787_Relay2.m.Vpu,SEL_787_Relay3.m.Vpu,SEL_787_Relay4.m.Vpu,SEL_787_Relay5.m.Vpu,SEL_787_Relay6.m.Vpu,SEL_787_Relay7.m.Vpu,SEL_787_Relay8.m.Vpu,SEL_787_Relay9.m.Vpu,SEL_787_Relay10.m.Vpu,SEL_787_Relay11.m.Vpu,SEL_787_Relay12.m.Vpu,SEL_787_Relay13.m.Vpu,SEL_787_Relay14.m.Vpu,SEL_787_Relay15.m.Vpu,SEL_787_Relay16.m.Vpu,SEL_787_Relay17.m.Vpu,SEL_787_Relay18.m.Vpu,SEL_787_Relay19.m.Vpu
  Bus Selector11 : BusSelector  OutputSignals=SEL_787_Relay1.m.P,SEL_787_Relay1.m.Q,SEL_787_Relay1.m.pf
  Bus Selector12 : BusSelector  OutputSignals=SEL_787_Relay13.m.P,SEL_787_Relay13.m.Q,SEL_787_Relay17.m.P
  Bus Selector13 : BusSelector  OutputSignals=SEL_787_Relay7.m.Vabc,SEL_787_Relay7.m.P,SEL_787_Relay7.m.Q,SEL_787_Relay8.m.Vabc,SEL_787_Relay8.m.P,SEL_787_Relay8.m.Q
  Bus Selector14 : BusSelector  OutputSignals=SEL_787_Relay1.m.status,SEL_787_Relay2.m.status,SEL_787_Relay3.m.status,SEL_787_Relay4.m.status,SEL_787_Relay5.m.status,SEL_787_Relay6.m.status,SEL_787_Relay7.m.status,SEL_787_Relay8.m.status,SEL_787_Relay9.m.status,SEL_787_Relay10.m.status,SEL_787_Relay11.m.status,SEL_787_Relay12.m.status,SEL_787_Relay13.m.status,SEL_787_Relay14.m.status,SEL_787_Relay15.m.status,SEL_787_Relay16.m.status,SEL_787_Relay17.m.status,SEL_787_Relay18.m.status,SEL_787_Relay19.m.status
  Gain{,1..6} (7 alike) : Gain  Gain=1/1000
  Gain7 : Gain  Gain=1/460
  Gain8 : Gain  Gain=1/13800
  Mux : Mux  Inputs=19
  Mux1 : Mux  Inputs=19
  Mux{2..5} (4 alike) : Mux  Inputs=2
  overall-scope : Scope  NumInputPorts=10
      settings: TimeRange=120  YMin=0~-15000~-1.2~-4500~-4500~0~-2~-500~-2~-500  YMax=1.2~15000~1.2~4500~1000~10~2~3000~2~4500  SaveName=ScopeData14
  wires:
  Mux2/1 -> overall-scope/2  "PCC_kW-kvar"
  Mux/1 -> overall-scope/1  "Vpu"
  Bus Selector11/3 -> overall-scope/3  "<pf>"
  Mux3/1 -> overall-scope/4  "Batt_kW_kvar"
  Gain1/1 -> overall-scope/5  "PV_kW"
  Mux1/1 -> overall-scope/6  "Status"
  Gain5/1 -> overall-scope/8  "G1_kW_kvar"
  Gain6/1 -> overall-scope/10  "G2_kW_kvar"
  Gain7/1 -> overall-scope/7  "G1_Vpu"
  Gain8/1 -> overall-scope/9  "G2_Vpu"
  Bus Selector13/6 -> Mux5/2  "<Q>"
  Bus Selector13/5 -> Mux5/1  "<P>"
  Mux5/1 -> Gain6/1
  Bus Selector13/4 -> Gain8/1  "<Vabc>"
  Mux4/1 -> Gain5/1
  Bus Selector13/3 -> Mux4/2  "<Q>"
  Bus Selector13/2 -> Mux4/1  "<P>"
  Bus Selector13/1 -> Gain7/1  "<Vabc>"
  Gain/1 -> Mux3/2  "Batt_kvar"
  Gain2/1 -> Mux3/1  "Batt_kW"
  Gain4/1 -> Mux2/2  "PCC_kvar"
  Gain3/1 -> Mux2/1  "PCC_kW"
  Bus Selector14/19 -> Mux1/19  "<status>"
  Bus Selector14/18 -> Mux1/18  "<status>"
  Bus Selector14/17 -> Mux1/17  "<status>"
  Bus Selector14/16 -> Mux1/16  "<status>"
  Bus Selector14/15 -> Mux1/15  "<status>"
  Bus Selector14/14 -> Mux1/14  "<status>"
  Bus Selector14/13 -> Mux1/13  "<status>"
  Bus Selector14/12 -> Mux1/12  "<status>"
  Bus Selector14/11 -> Mux1/11  "<status>"
  Bus Selector14/10 -> Mux1/10  "<status>"
  Bus Selector14/9 -> Mux1/9  "<status>"
  Bus Selector14/8 -> Mux1/8  "<status>"
  Bus Selector14/7 -> Mux1/7  "<status>"
  Bus Selector14/6 -> Mux1/6  "<status>"
  Bus Selector14/5 -> Mux1/5  "<status>"
  Bus Selector14/4 -> Mux1/4  "<status>"
  Bus Selector14/3 -> Mux1/3  "<status>"
  Bus Selector14/2 -> Mux1/2  "<status>"
  Bus Selector14/1 -> Mux1/1  "<status>"
  Bus Selector12/3 -> Gain1/1  "<P>"
  Bus Selector12/2 -> Gain/1  "<Q>"
  Bus Selector12/1 -> Gain2/1  "<P>"
  Bus Selector11/2 -> Gain4/1  "<Q>"
  Bus Selector11/1 -> Gain3/1  "<P>"
  Bus Selector10/19 -> Mux/19  "<Vpu>"
  Bus Selector10/18 -> Mux/18  "<Vpu>"
  Bus Selector10/17 -> Mux/17  "<Vpu>"
  Bus Selector10/16 -> Mux/16  "<Vpu>"
  Bus Selector10/15 -> Mux/15  "<Vpu>"
  Bus Selector10/14 -> Mux/14  "<Vpu>"
  Bus Selector10/13 -> Mux/13  "<Vpu>"
  Bus Selector10/12 -> Mux/12  "<Vpu>"
  Bus Selector10/11 -> Mux/11  "<Vpu>"
  Bus Selector10/10 -> Mux/10  "<Vpu>"
  Bus Selector10/9 -> Mux/9  "<Vpu>"
  Bus Selector10/8 -> Mux/8  "<Vpu>"
  Bus Selector10/7 -> Mux/7  "<Vpu>"
  Bus Selector10/6 -> Mux/6  "<Vpu>"
  Bus Selector10/5 -> Mux/5  "<Vpu>"
  Bus Selector10/4 -> Mux/4  "<Vpu>"
  Bus Selector10/3 -> Mux/3  "<Vpu>"
  Bus Selector10/2 -> Mux/2  "<Vpu>"
  Bus Selector10/1 -> Mux/1  "<Vpu>"
  ms/1 -> Bus Selector13/1, Bus Selector14/1, Bus Selector12/1, Bus Selector11/1, Bus Selector10/1

== system MODEL_FULL_SYSTEM_MUTUAL/SM_Master/Gen_initial_condition_1MVA ==
  1 - PQ 2 - PV 3 - VF : Constant
  Bus Creator : BusCreator  Inputs=6
  DONOTCHANGE : Constant
  F : simulink/Math Operations/Slider Gain  low=0  gain=1  high=1
  P : simulink/Math Operations/Slider Gain  low=0  gain=0.8  high=1
  Q : simulink/Math Operations/Slider Gain  low=0  gain=0.2  high=0.5
  V : simulink/Math Operations/Slider Gain  low=0  gain=1  high=1
  e : Constant  Value=0
  S : Outport
  wires:
  1 - PQ 2 - PV 3 - VF/1 -> Bus Creator/5  "Mode"
  F/1 -> Bus Creator/4  "F"
  V/1 -> Bus Creator/3  "V"
  Q/1 -> Bus Creator/2  "Q"
  P/1 -> Bus Creator/1  "P"
  Bus Creator/1 -> S/1
  DONOTCHANGE/1 -> F/1, V/1, Q/1, P/1
  e/1 -> Bus Creator/6  "Enable"

== system MODEL_FULL_SYSTEM_MUTUAL/SM_Master/Gen_initial_condition_4MVA ==
  1 - PQ 2 - PV 3 - VF : Constant
  Bus Creator : BusCreator  Inputs=6
  DONOTCHANGE : Constant
  F : simulink/Math Operations/Slider Gain  low=0  gain=1  high=1
  P : simulink/Math Operations/Slider Gain  low=0  gain=0.9  high=1
  Q : simulink/Math Operations/Slider Gain  low=0  gain=0.2  high=0.5
  V : simulink/Math Operations/Slider Gain  low=0  gain=1  high=1
  e : Constant  Value=0
  S : Outport
  wires:
  1 - PQ 2 - PV 3 - VF/1 -> Bus Creator/5  "Mode"
  F/1 -> Bus Creator/4  "F"
  V/1 -> Bus Creator/3  "V"
  Q/1 -> Bus Creator/2  "Q"
  P/1 -> Bus Creator/1  "P"
  Bus Creator/1 -> S/1
  DONOTCHANGE/1 -> F/1, V/1, Q/1, P/1
  e/1 -> Bus Creator/6  "Enable"

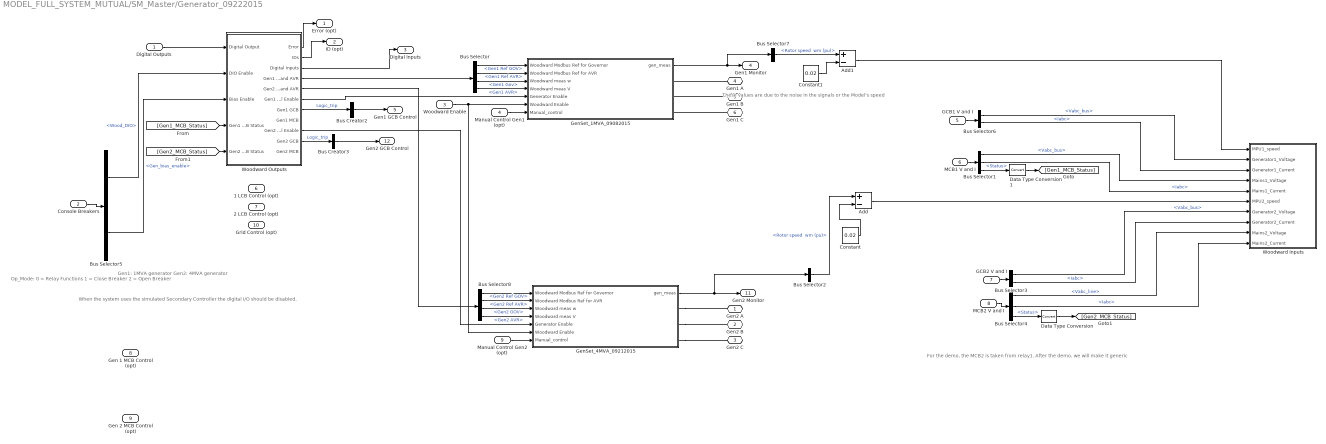
== system MODEL_FULL_SYSTEM_MUTUAL/SM_Master/Generator_09222015 ==
  note: Op_Mode:
      | 0 = Relay Functions
      | 1 = Close Breaker
      | 2 = Open Breaker
  note: These values are due to
      | the noise in the signals
      | or the Model's speed
  note: Gen1: 1MVA generator
      | Gen2: 4MVA generator
  note: When the system uses the simulated
      | Secondary Controller the digital I/O
      | should be disabled.
  note: For the demo, the MCB2  is taken from relay1.
      |  After the demo, we will make it generic
  Digital Outputs : Inport
  Console Breakers : Inport  Port=2
  Woodward Enable : Inport  Port=3
  Manual Control Gen1 (opt) : Inport  Port=4
  GCB1 V and I : Inport  Port=5
  MCB1 V and I : Inport  Port=6
  GCB2 V and I : Inport  Port=7
  MCB2 V and I : Inport  Port=8
  Manual Control Gen2 (opt) : Inport  Port=9
  Add : Sum  Inputs=+-
  Add1 : Sum  Inputs=+-
  Bus Creator2 : BusCreator  Inputs=1
  Bus Creator3 : BusCreator  Inputs=1
  Bus Selector : BusSelector  OutputSignals=Gen1 Ref GOV,Gen1 Ref AVR,Gen1 Gov,Gen1 AVR
  Bus Selector1 : BusSelector  OutputSignals=Vabc_bus,Iabc,Status
  Bus Selector2 : BusSelector  OutputSignals="w.w.Rotor speed  wm (pu)"
  Bus Selector3 : BusSelector  OutputSignals=Vabc_bus,Iabc
  Bus Selector4 : BusSelector  OutputSignals=Vabc_line,Iabc,Status
  Bus Selector5 : BusSelector  OutputSignals=Wood_DIO,Gen_bias_enable
  Bus Selector6 : BusSelector  OutputSignals=Vabc_bus,Iabc
  Bus Selector7 : BusSelector  OutputSignals="w.w.Rotor speed  wm (pu)"
  Bus Selector8 : BusSelector  OutputSignals=Gen2 Ref GOV,Gen2 Ref AVR,Gen2 GOV,Gen2 AVR
  Constant : Constant  Value=0.02
  Constant1 : Constant  Value=0.02
  Data Type Conversion : DataTypeConversion
  Data Type Conversion1 : DataTypeConversion
  GenSet_1MVA_09082015 : Subsystem  mask(Gen-Set with simulated control modes){control_mode=1}
      mask prompts: control_mode "Control Mode [0 => Sim. 1 => Wood.]"
      mask help:
      | This Gen-Set block allows the user to indicate the control mode of the generator. The available control modes are: (1) PQ, (2) PV, and (3) VF.
      | The input values to the block will be applied according to the selected control mode.
      | For example, if PQ mode is selected, the controller will only work based on P_ref and Q_ref ignoring values of other inputs to the block.
  GenSet_4MVA_09212015 : Subsystem  mask(Gen-Set with simulated control modes){control_mode=1}
      mask prompts: control_mode "Control Mode [0 => Sim. 1 => Wood.]"
      mask help:
      | This Gen-Set block allows the user to indicate the control mode of the generator. The available control modes are: (1) PQ, (2) PV, and (3) VF.
      | The input values to the block will be applied according to the selected control mode.
      | For example, if PQ mode is selected, the controller will only work based on P_ref and Q_ref ignoring values of other inputs to the block.
  Woodward Inputs : Subsystem
  Woodward Outputs : Subsystem
  Gen2 A : PMIOPort  Port=1  Side=Right
  Gen2 B : PMIOPort  Port=2  Side=Right
  Gen2 C : PMIOPort  Port=3  Side=Right
  Gen1 A : PMIOPort  Port=4  Side=Right
  Gen1 B : PMIOPort  Port=5  Side=Right
  Gen1 C : PMIOPort  Port=6  Side=Right
  Error (opt) : Outport
  ID (opt) : Outport  Port=2
  Digital Inputs : Outport  Port=3
  Gen1 Monitor : Outport  Port=4
  Gen1 GCB Control : Outport  Port=5
  1 LCB Control (opt) : Outport  Port=6
  2 LCB Control (opt) : Outport  Port=7
  Gen 1 MCB Control (opt) : Outport  Port=8
  Gen 2 MCB Control (opt) : Outport  Port=9
  Grid Control (opt) : Outport  Port=10
  Gen2 Monitor : Outport  Port=11
  Gen2 GCB Control : Outport  Port=12
  wires:
  GenSet_1MVA_09082015/1(gen_meas) -> Bus Selector7/1, Gen1 Monitor/1
  Bus Selector5/1 -> Woodward Outputs/2(DIO Enable)  "<Wood_DIO>"
  Manual Control Gen1 (opt)/1 -> GenSet_1MVA_09082015/7(Manual_control)
  Bus Selector5/2 -> Woodward Outputs/3(Bias Enable)  "<Gen_bias_enable>"
  Bus Selector7/1 -> Add1/1  "<Rotor speed  wm (pu)>"
  Woodward Outputs/1(Error) -> Error (opt)/1
  Woodward Outputs/2(IDs) -> ID (opt)/1
  Woodward Outputs/3(Digital Inputs) -> Digital Inputs/1
  Woodward Enable/1 -> GenSet_1MVA_09082015/6(Woodward Enable), GenSet_4MVA_09212015/6(Woodward Enable)
  Woodward Outputs/6(Gen1 Fuel Enable) -> GenSet_1MVA_09082015/5(Generator Enable)
  Digital Outputs/1 -> Woodward Outputs/1(Digital Output)
  GCB1 V and I/1 -> Bus Selector6/1
  Woodward Outputs/7(Gen1 GCB) -> Bus Creator2/1  "Logic_trip"
  Console Breakers/1 -> Bus Selector5/1
  MCB1 V and I/1 -> Bus Selector1/1
  GCB2 V and I/1 -> Bus Selector3/1
  MCB2 V and I/1 -> Bus Selector4/1
  GenSet_4MVA_09212015/1(gen_meas) -> Gen2 Monitor/1, Bus Selector2/1
  Bus Selector2/1 -> Add/1  "<Rotor speed  wm (pu)>"
  Woodward Outputs/4(Gen1 Gov and AVR) -> Bus Selector/1
  Bus Selector/1 -> GenSet_1MVA_09082015/1(Woodward Modbus Ref for Governor)  "<Gen1 Ref GOV>"
  Bus Selector/2 -> GenSet_1MVA_09082015/2(Woodward Modbus Ref for AVR)  "<Gen1 Ref AVR>"
  Bus Selector/3 -> GenSet_1MVA_09082015/3(Woodward meas w)  "<Gen1 Gov>"
  Bus Selector/4 -> GenSet_1MVA_09082015/4(Woodward meas V)  "<Gen1 AVR>"
  Woodward Outputs/5(Gen2 Gov and AVR) -> Bus Selector8/1
  Bus Selector8/1 -> GenSet_4MVA_09212015/1(Woodward Modbus Ref for Governor)  "<Gen2 Ref GOV>"
  Bus Selector8/2 -> GenSet_4MVA_09212015/2(Woodward Modbus Ref for AVR)  "<Gen2 Ref AVR>"
  Bus Selector8/3 -> GenSet_4MVA_09212015/3(Woodward meas w)  "<Gen2 GOV>"
  Bus Selector8/4 -> GenSet_4MVA_09212015/4(Woodward meas V)  "<Gen2 AVR>"
  Manual Control Gen2 (opt)/1 -> GenSet_4MVA_09212015/7(Manual_control)
  Woodward Outputs/9(Gen2 Fuel Enable) -> GenSet_4MVA_09212015/5(Generator Enable)
  Woodward Outputs/10(Gen2 GCB) -> Bus Creator3/1  "Logic_trip"
  Add/1 -> Woodward Inputs/6(MPU2_speed)
  Constant/1 -> Add/2
  Bus Selector1/3 -> Data Type Conversion1/1  "<Status>"
  Bus Selector4/3 -> Data Type Conversion/1  "<Status>"
  [Gen1_MCB_Status] -> Woodward Outputs/4(Gen1 MCB Status)
  [Gen2_MCB_Status] -> Woodward Outputs/5(Gen2 MCB Status)
  Constant1/1 -> Add1/2
  Add1/1 -> Woodward Inputs/1(MPU1_speed)
  Bus Selector3/1 -> Woodward Inputs/7(Generator2_Voltage)  "<Vabc_bus>"
  Bus Selector3/2 -> Woodward Inputs/8(Generator2_Current)  "<Iabc>"
  Bus Selector4/1 -> Woodward Inputs/9(Mains2_Voltage)  "<Vabc_line>"
  Bus Selector4/2 -> Woodward Inputs/10(Mains2_Current)  "<Iabc>"
  Bus Selector6/1 -> Woodward Inputs/2(Generator1_Voltage)  "<Vabc_bus>"
  Bus Selector6/2 -> Woodward Inputs/3(Generator1_Current)  "<Iabc>"
  Bus Selector1/1 -> Woodward Inputs/4(Mains1_Voltage)  "<Vabc_bus>"
  Bus Selector1/2 -> Woodward Inputs/5(Mains1_Current)  "<Iabc>"
  Bus Creator3/1 -> Gen2 GCB Control/1
  Bus Creator2/1 -> Gen1 GCB Control/1
  Data Type Conversion/1 -> [Gen2_MCB_Status]
  Data Type Conversion1/1 -> [Gen1_MCB_Status]
  connections:
  Gen1 A/RConn1 -- GenSet_1MVA_09082015/RConn1
  Gen1 B/RConn1 -- GenSet_1MVA_09082015/RConn2
  Gen1 C/RConn1 -- GenSet_1MVA_09082015/RConn3
  GenSet_4MVA_09212015/RConn1 -- Gen2 A/RConn1
  GenSet_4MVA_09212015/RConn2 -- Gen2 B/RConn1
  GenSet_4MVA_09212015/RConn3 -- Gen2 C/RConn1

== system MODEL_FULL_SYSTEM_MUTUAL/SS_Slave/BATT_MODBUS ==
  MSMTS : Inport
  faults : Inport  Port=2
  1 - Enable 0 - Disable1 : Constant  Value=200
  1 - Enable 0 - Disable2 : Constant  Value=500
  1 - Enable 0 - Disable3 : Constant  Value=0
  Bus Creator : BusCreator  Inputs=3
  Bus Creator1 : BusCreator  Inputs=3
  Bus Creator2 : BusCreator
  Bus Selector : BusSelector  OutputSignals=Capacity (signal 2)
  Data Type Conversion : DataTypeConversion
  Data Type Conversion1 : DataTypeConversion
  Demux : Demux
  Digital Clock : DigitalClock  SampleTime=Ts
  Gain1 : Gain  Gain=100
  MATLAB Function : MATLAB Function  TreatAsAtomicUnit=on
  MATLAB Function1 : MATLAB Function  TreatAsAtomicUnit=on
  Math Function : Math  Operator=mod  SaturateOnIntegerOverflow=on
  Memory : Memory
  Memory1 : Memory
  Modbus device : rtio_generic_modbus/Modbus device  conf_name=batt_slave_cfg.opal  conf_name_mask=batt_slave_cfg.xls  sample_time=Ts
  Switch1 : Switch  Criteria=u2 > Threshold
  Switch2 : Switch  Criteria=u2 > Threshold
  Switch3 : Switch  Criteria=u2 > Threshold
  bitwise_faults : Subsystem
  simulation time limit : Constant  Value=900
  Batt_control : Outport
  fm_mb : Outport  Port=2
  faults_bitwise : Outport  Port=3
  wires:
  Modbus device/2 -> Demux/1
  1 - Enable 0 - Disable1/1 -> Switch1/3
  1 - Enable 0 - Disable2/1 -> Switch2/3
  1 - Enable 0 - Disable3/1 -> Switch3/3
  Demux/2 -> MATLAB Function/1(x)  "reg1"
  Demux/3 -> MATLAB Function1/1(x)  "reg2"
  Demux/4 -> Switch3/1, Bus Creator2/4  "cmd_reg4_enable"
  Demux/1 -> Switch1/2, Switch2/2, Switch3/2, Bus Creator2/1  "cmd_reg0"
  Switch1/1 -> Bus Creator/1  "kvar"
  Switch2/1 -> Bus Creator/2  "kW"
  Switch3/1 -> Bus Creator/3  "Enable"
  Bus Creator/1 -> Batt_control/1
  MSMTS/1 -> Bus Selector/1
  Bus Selector/1 -> Data Type Conversion/1  "<Capacity (signal 2)>"
  Data Type Conversion/1 -> Gain1/1
  Bus Creator1/1 -> Modbus device/4
  Gain1/1 -> Bus Creator1/2
  Bus Creator2/1 -> fm_mb/1
  bitwise_faults/1(to_mb) -> Memory/1
  faults/1 -> bitwise_faults/1(batt_fault)
  Memory/1 -> Bus Creator1/1, faults_bitwise/1
  MATLAB Function1/1(y) -> Switch2/1, Bus Creator2/3  "cmd_reg2_kw"
  MATLAB Function/1(y) -> Switch1/1, Bus Creator2/2  "cmd_reg1_kvar"
  Digital Clock/1 -> Math Function/1
  simulation time limit/1 -> Math Function/2
  Math Function/1 -> Data Type Conversion1/1
  Data Type Conversion1/1 -> Memory1/1
  Memory1/1 -> Bus Creator1/3

== system MODEL_FULL_SYSTEM_MUTUAL/SS_Slave/Data to record with OpWriteFile ==
  note: data mapping to output vector:
      | field_1 : time
      | field_2 : PCC power factor
      | field_3-21 : kw
      | field_22-40 : kvar
      | field_41-59 : Vpu
      | field_60-65 : frequency
      | field_66-84 : relay status as bitwise
      | field_85 : battery SoC
      | field_86 : batt cmd reg 0
      | field_87 : batt cmd reg 1 - kvar
      | field_88 : batt cmd reg 2 - kw
      | field_89 : batt cmd reg 3 - enable
      | field_90 : battery faults as bitwise
      | field_91 : gen_1MVA gal_per_hr
      | field_92 : gen_4MVA gal_per_hr
  note: Relay function status as bitwise:
      | R25-R27-R50-R51-R59-Reset
  note: The signals will appear in the mat file in the same order that are being vectorized
  ms : Inport
  batt : Inport  Port=2
  gen : Inport  Port=3
  Bus Selector1 : BusSelector  OutputSignals=SEL_787_Relay1.m.P,SEL_787_Relay2.m.P,SEL_787_Relay3.m.P,SEL_787_Relay4.m.P,SEL_787_Relay5.m.P,SEL_787_Relay6.m.P,SEL_787_Relay7.m.P,SEL_787_Relay8.m.P,SEL_787_Relay9.m.P,SEL_787_Relay10.m.P,SEL_787_Relay11.m.P,SEL_787_Relay12.m.P,SEL_787_Relay13.m.P,SEL_787_Relay14.m.P,SEL_787_Relay15.m.P,SEL_787_Relay16.m.P,SEL_787_Relay17.m.P,SEL_787_Relay18.m.P,SEL_787_Relay19.m.P
  Bus Selector2 : BusSelector  OutputSignals=SEL_787_Relay1.m.Q,SEL_787_Relay2.m.Q,SEL_787_Relay3.m.Q,SEL_787_Relay4.m.Q,SEL_787_Relay5.m.Q,SEL_787_Relay6.m.Q,SEL_787_Relay7.m.Q,SEL_787_Relay8.m.Q,SEL_787_Relay9.m.Q,SEL_787_Relay10.m.Q,SEL_787_Relay11.m.Q,SEL_787_Relay12.m.Q,SEL_787_Relay13.m.Q,SEL_787_Relay14.m.Q,SEL_787_Relay15.m.Q,SEL_787_Relay16.m.Q,SEL_787_Relay17.m.Q,SEL_787_Relay18.m.Q,SEL_787_Relay19.m.Q
  Bus Selector3 : BusSelector  OutputSignals=SEL_787_Relay1.m.Vpu,SEL_787_Relay2.m.Vpu,SEL_787_Relay3.m.Vpu,SEL_787_Relay4.m.Vpu,SEL_787_Relay5.m.Vpu,SEL_787_Relay6.m.Vpu,SEL_787_Relay7.m.Vpu,SEL_787_Relay8.m.Vpu,SEL_787_Relay9.m.Vpu,SEL_787_Relay10.m.Vpu,SEL_787_Relay11.m.Vpu,SEL_787_Relay12.m.Vpu,SEL_787_Relay13.m.Vpu,SEL_787_Relay14.m.Vpu,SEL_787_Relay15.m.Vpu,SEL_787_Relay16.m.Vpu,SEL_787_Relay17.m.Vpu,SEL_787_Relay18.m.Vpu,SEL_787_Relay19.m.Vpu
  Bus Selector4 : BusSelector  OutputSignals=SEL_787_Relay1.m.freq,SEL_787_Relay3.m.freq,SEL_787_Relay7.m.freq,SEL_787_Relay8.m.freq,SEL_787_Relay13.m.freq,SEL_787_Relay17.m.freq
  Bus Selector5 : BusSelector  OutputSignals=SEL_787_Relay1.m.status,SEL_787_Relay2.m.status,SEL_787_Relay3.m.status,SEL_787_Relay4.m.status,SEL_787_Relay5.m.status,SEL_787_Relay6.m.status,SEL_787_Relay7.m.status,SEL_787_Relay8.m.status,SEL_787_Relay9.m.status,SEL_787_Relay10.m.status,SEL_787_Relay11.m.status,SEL_787_Relay12.m.status,SEL_787_Relay13.m.status,SEL_787_Relay14.m.status,SEL_787_Relay15.m.status,SEL_787_Relay16.m.status,SEL_787_Relay17.m.status,SEL_787_Relay18.m.status,SEL_787_Relay19.m.status
  Bus Selector6 : BusSelector  OutputSignals=Capacity.Capacity (signal 2),controller_cmds.cmd_reg0,controller_cmds.cmd_reg1_kvar,controller_cmds.cmd_reg2_kw,controller_cmds.cmd_reg4_enable,faults
  Bus Selector7 : BusSelector  OutputSignals=SEL_787_Relay1.m.pf
  Bus Selector8 : BusSelector  OutputSignals=gal_per_hr_1MVA,gal_per_hr_4MVA
  Gain2 : Gain  Gain=1/1000
  Gain3 : Gain  Gain=1/1000
  Mux{1..3,5} (4 alike) : Mux  Inputs=19
  Mux4 : Mux  Inputs=6
  Mux6 : Mux  Inputs=6
  Mux7 : Mux  Inputs=8
  Mux8 : Mux  Inputs=2
  to OpWriteFile : Outport
  wires:
  ms/1 -> Bus Selector1/1, Bus Selector2/1, Bus Selector3/1, Bus Selector4/1, Bus Selector5/1, Bus Selector7/1
  Bus Selector1/1 -> Mux1/1  "<P>"
  Bus Selector1/2 -> Mux1/2  "<P>"
  Bus Selector1/3 -> Mux1/3  "<P>"
  Bus Selector1/4 -> Mux1/4  "<P>"
  Bus Selector1/5 -> Mux1/5  "<P>"
  Bus Selector1/6 -> Mux1/6  "<P>"
  Bus Selector1/7 -> Mux1/7  "<P>"
  Bus Selector1/8 -> Mux1/8  "<P>"
  Bus Selector1/9 -> Mux1/9  "<P>"
  Bus Selector1/10 -> Mux1/10  "<P>"
  Bus Selector1/11 -> Mux1/11  "<P>"
  Bus Selector1/12 -> Mux1/12  "<P>"
  Bus Selector1/13 -> Mux1/13  "<P>"
  Bus Selector1/14 -> Mux1/14  "<P>"
  Bus Selector1/15 -> Mux1/15  "<P>"
  Bus Selector1/16 -> Mux1/16  "<P>"
  Bus Selector1/17 -> Mux1/17  "<P>"
  Bus Selector1/18 -> Mux1/18  "<P>"
  Bus Selector1/19 -> Mux1/19  "<P>"
  Mux1/1 -> Gain2/1
  Gain2/1 -> [kW]  "kW"
  Bus Selector2/1 -> Mux2/1  "<Q>"
  Bus Selector2/2 -> Mux2/2  "<Q>"
  Bus Selector2/3 -> Mux2/3  "<Q>"
  Bus Selector2/4 -> Mux2/4  "<Q>"
  Bus Selector2/5 -> Mux2/5  "<Q>"
  Bus Selector2/6 -> Mux2/6  "<Q>"
  Bus Selector2/7 -> Mux2/7  "<Q>"
  Bus Selector2/8 -> Mux2/8  "<Q>"
  Bus Selector2/9 -> Mux2/9  "<Q>"
  Bus Selector2/10 -> Mux2/10  "<Q>"
  Bus Selector2/11 -> Mux2/11  "<Q>"
  Bus Selector2/12 -> Mux2/12  "<Q>"
  Bus Selector2/13 -> Mux2/13  "<Q>"
  Bus Selector2/14 -> Mux2/14  "<Q>"
  Bus Selector2/15 -> Mux2/15  "<Q>"
  Bus Selector2/16 -> Mux2/16  "<Q>"
  Bus Selector2/17 -> Mux2/17  "<Q>"
  Bus Selector2/18 -> Mux2/18  "<Q>"
  Bus Selector2/19 -> Mux2/19  "<Q>"
  Mux2/1 -> Gain3/1
  Gain3/1 -> [kvar]  "kvar"
  Bus Selector3/1 -> Mux3/1  "<Vpu>"
  Bus Selector3/2 -> Mux3/2  "<Vpu>"
  Bus Selector3/3 -> Mux3/3  "<Vpu>"
  Bus Selector3/4 -> Mux3/4  "<Vpu>"
  Bus Selector3/5 -> Mux3/5  "<Vpu>"
  Bus Selector3/6 -> Mux3/6  "<Vpu>"
  Bus Selector3/7 -> Mux3/7  "<Vpu>"
  Bus Selector3/8 -> Mux3/8  "<Vpu>"
  Bus Selector3/9 -> Mux3/9  "<Vpu>"
  Bus Selector3/10 -> Mux3/10  "<Vpu>"
  Bus Selector3/11 -> Mux3/11  "<Vpu>"
  Bus Selector3/12 -> Mux3/12  "<Vpu>"
  Bus Selector3/13 -> Mux3/13  "<Vpu>"
  Bus Selector3/14 -> Mux3/14  "<Vpu>"
  Bus Selector3/15 -> Mux3/15  "<Vpu>"
  Bus Selector3/16 -> Mux3/16  "<Vpu>"
  Bus Selector3/17 -> Mux3/17  "<Vpu>"
  Bus Selector3/18 -> Mux3/18  "<Vpu>"
  Bus Selector3/19 -> Mux3/19  "<Vpu>"
  Mux3/1 -> [Vpu]
  Mux4/1 -> [freq]  "Hz"
  Mux5/1 -> [status]
  Bus Selector5/1 -> Mux5/1  "<status>"
  Bus Selector5/2 -> Mux5/2  "<status>"
  Bus Selector5/3 -> Mux5/3  "<status>"
  Bus Selector5/4 -> Mux5/4  "<status>"
  Bus Selector5/5 -> Mux5/5  "<status>"
  Bus Selector5/6 -> Mux5/6  "<status>"
  Bus Selector5/7 -> Mux5/7  "<status>"
  Bus Selector5/8 -> Mux5/8  "<status>"
  Bus Selector5/9 -> Mux5/9  "<status>"
  Bus Selector5/10 -> Mux5/10  "<status>"
  Bus Selector5/11 -> Mux5/11  "<status>"
  Bus Selector5/12 -> Mux5/12  "<status>"
  Bus Selector5/13 -> Mux5/13  "<status>"
  Bus Selector5/14 -> Mux5/14  "<status>"
  Bus Selector5/15 -> Mux5/15  "<status>"
  Bus Selector5/16 -> Mux5/16  "<status>"
  Bus Selector5/17 -> Mux5/17  "<status>"
  Bus Selector5/18 -> Mux5/18  "<status>"
  Bus Selector5/19 -> Mux5/19  "<status>"
  batt/1 -> Bus Selector6/1
  Bus Selector7/1 -> [pf]  "<pf>"
  Bus Selector6/1 -> Mux6/1  "<Capacity (signal 2)>"
  Bus Selector6/2 -> Mux6/2  "<cmd_reg0>"
  Bus Selector6/3 -> Mux6/3  "<cmd_reg1_kvar>"
  Bus Selector6/4 -> Mux6/4  "<cmd_reg2_kw>"
  Bus Selector6/5 -> Mux6/5  "<cmd_reg4_enable>"
  Bus Selector6/6 -> Mux6/6  "<faults>"
  Mux6/1 -> [batt_meas]
  [pf] -> Mux7/1
  [kW] -> Mux7/2
  [kvar] -> Mux7/3
  [Vpu] -> Mux7/4
  [freq] -> Mux7/5
  [status] -> Mux7/6
  [batt_meas] -> Mux7/7
  Mux7/1 -> to OpWriteFile/1
  Bus Selector4/1 -> Mux4/1  "<freq>"
  Bus Selector4/2 -> Mux4/2  "<freq>"
  Bus Selector4/3 -> Mux4/3  "<freq>"
  Bus Selector4/4 -> Mux4/4  "<freq>"
  Bus Selector4/5 -> Mux4/5  "<freq>"
  Bus Selector4/6 -> Mux4/6  "<freq>"
  Mux8/1 -> [gen_meas]
  [gen_meas] -> Mux7/8
  gen/1 -> Bus Selector8/1
  Bus Selector8/1 -> Mux8/1  "<gal_per_hr_1MVA>"
  Bus Selector8/2 -> Mux8/2  "<gal_per_hr_4MVA>"
